simulink model "t8_videoclase3_beta"  (R2022b)
settings: Solver=FixedStepAuto  StartTime=0.0  StopTime=10  FixedStep=.01  RelTol=1e-3
model workspace (MATLAB code in the model file):
  | v0=30;
  | theta0=pi/6;
settings Model: Creator=scpmoxxa  LastModifiedBy=scpmoxxa

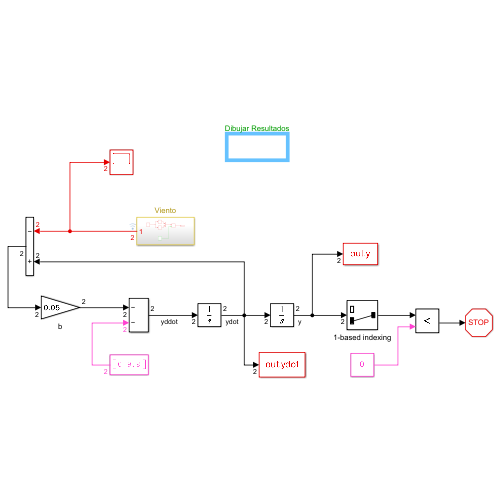
[thumbnail: Simulink's stored preview of the top-level diagram]
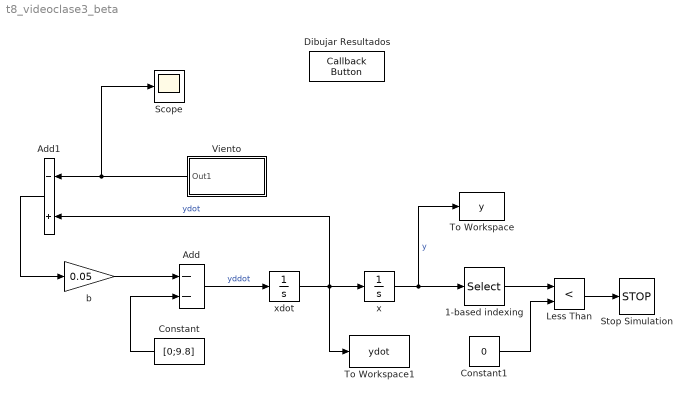
== system t8_videoclase3_beta ==
  1-based indexing : Selector  InputPortWidth=2  IndexOptions=Index vector (dialog)  Indices=2  OutputSizes=1
  Add : Sum  Inputs=--
  Add1 : Sum  Inputs=-+
  Constant : Constant  Value=[0;9.8]
  Constant1 : Constant  Value=0
  Dibujar Resultados : CallbackButton  ButtonText=Plot results
      settings: ClickFcn=|
      | %plot results
      | close all
      | 
      | t=out.tout;
      | 
      | figure(1)
      | subplot(2,2,1)
      | plot(t,out.y)
      | xlabel('t')
      | ylabel('Posicion')
      | legend('x','y')
      | 
      | subplot(2,2,3)
      | plot(t,out.ydot)
      | xlabel('t')
      | ylabel('Velocidad')
      | legend('Vx','Vy')
      | 
      | subplot(2,2,[2,4])
      | plot(out.y(:,1),out.y(:,2))
      | xlabel('x')
      | ylabel('y')
  Less Than : RelationalOperator  Operator=<  OutDataTypeStr=boolean  RndMeth=Simplest  InputSameDT=off
  Scope : Scope
  Stop Simulation : Stop
  To Workspace : ToWorkspace  VariableName=y  SampleTime=-1
  To Workspace1 : ToWorkspace  VariableName=ydot  SampleTime=-1
  Viento : Subsystem
  b : Gain  Gain=0.05
  x : Integrator  InitialCondition=[0;20]
  xdot : Integrator  InitialCondition=[v0*cos(theta0);v0*sin(theta0)]
  wires:
  Constant1/1 -> Less Than/2
  x/1 -> 1-based indexing/1, To Workspace/1  "y"
  Less Than/1 -> Stop Simulation/1
  Add/1 -> xdot/1  "yddot"
  xdot/1 -> Add1/2, To Workspace1/1, x/1  "ydot"
  1-based indexing/1 -> Less Than/1
  Constant/1 -> Add/2
  b/1 -> Add/1
  Viento/1(Out1) -> Scope/1, Add1/1
  Add1/1 -> b/1

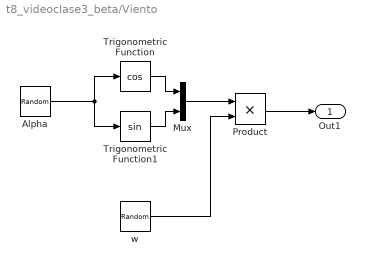
== system t8_videoclase3_beta/Viento ==
  Alpha : RandomNumber  Mean=pi  Variance=pi/10  Seed=randi(1e6)  SampleTime=0.01
  Mux : Mux  Inputs=2
  Product : Product
  Trigonometric Function : Trigonometry  Operator=cos
  Trigonometric Function1 : Trigonometry
  w : RandomNumber  Mean=v0/2  Variance=5  Seed=randi(1e6)  SampleTime=0.2
  Out1 : Outport
  wires:
  Trigonometric Function/1 -> Mux/1
  Alpha/1 -> Trigonometric Function/1, Trigonometric Function1/1
  w/1 -> Product/2
  Mux/1 -> Product/1
  Trigonometric Function1/1 -> Mux/2
  Product/1 -> Out1/1
